simulink model "Generated_Trajectory_Linear_System"  (R2020b)
settings: Solver=VariableStepAuto  StartTime=0.0  StopTime=t_sim  RelTol=1e-3
undefined symbols (not defined in the file): A1_sim, B1_sim, Beta0Vec1_sim, OL_Traj_Gain, omega_sim, r_sim
settings Model: Creator=domin  LastModifiedBy=domin

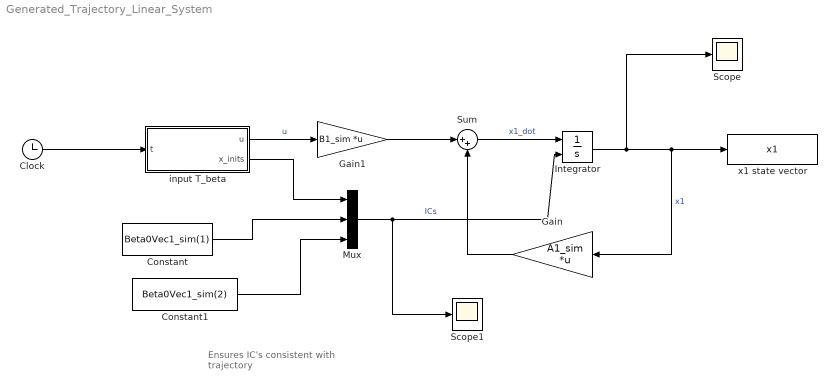
== system Generated_Trajectory_Linear_System ==
  note: Ensures IC's consistent with trajectory
  Clock : Clock
  Constant : Constant  Value=Beta0Vec1_sim(1)
  Constant1 : Constant  Value=Beta0Vec1_sim(2)
  Gain : Gain  Gain=A1_sim  Multiplication=Matrix(K*u)
  Gain1 : Gain  Gain=B1_sim  Multiplication=Matrix(K*u)
  Integrator : Integrator  InitialConditionSource=external
  Mux : Mux  Inputs=3
  Scope : Scope
  Scope1 : Scope
  Sum : Sum  Inputs=|++
  input T_beta : Subsystem
  x1 state vector : ToWorkspace  VariableName=x1  SampleTime=-1
  wires:
  Clock/1 -> input T_beta/1(t)
  Sum/1 -> Integrator/1  "x1_dot"
  Integrator/1 -> Scope/1, Gain/1, x1 state vector/1  "x1"
  input T_beta/1(u) -> Gain1/1  "u"
  Gain1/1 -> Sum/1
  Gain/1 -> Sum/2
  Constant1/1 -> Mux/3
  Constant/1 -> Mux/2
  input T_beta/2(x_inits) -> Mux/1
  Mux/1 -> Scope1/1, Integrator/2  "ICs"

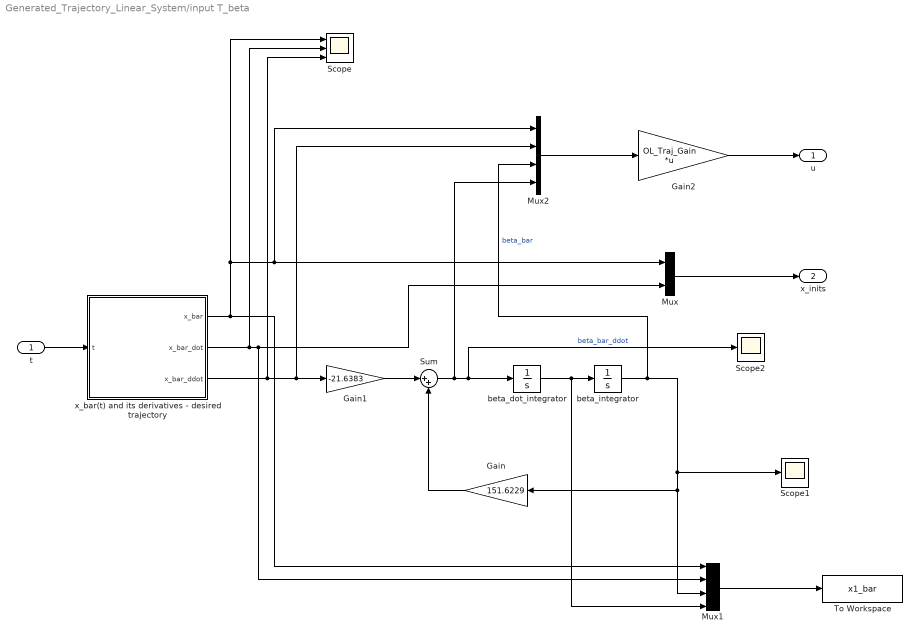
== system Generated_Trajectory_Linear_System/input T_beta ==
  t : Inport
  Gain : Gain  Gain=151.6229
  Gain1 : Gain  Gain=-21.6383
  Gain2 : Gain  Gain=OL_Traj_Gain  Multiplication=Matrix(K*u)
  Mux : Mux  Inputs=2
  Mux1 : Mux
  Mux2 : Mux
  Scope : Scope  NumInputPorts=3
  Scope1 : Scope
  Scope2 : Scope
  Sum : Sum  Inputs=|++
  To Workspace : ToWorkspace  VariableName=x1_bar  SampleTime=-1
  beta_dot_integrator : Integrator  InitialCondition=Beta0Vec1_sim(2)
  beta_integrator : Integrator  InitialCondition=Beta0Vec1_sim(1)
  x_bar(t) and its derivatives - desired trajectory : MATLAB Function  TreatAsAtomicUnit=on
  u : Outport
  x_inits : Outport  Port=2
  wires:
  t/1 -> x_bar(t) and its derivatives - desired trajectory/1(t)
  Sum/1 -> Mux2/4, Scope2/1, beta_dot_integrator/1  "beta_bar_ddot"
  beta_dot_integrator/1 -> Mux1/4, beta_integrator/1
  beta_integrator/1 -> Mux2/3, Mux1/3, Gain/1, Scope1/1  "beta_bar"
  Gain/1 -> Sum/2
  x_bar(t) and its derivatives - desired trajectory/3(x_bar_ddot) -> Scope/3, Mux2/2, Gain1/1
  Gain1/1 -> Sum/1
  x_bar(t) and its derivatives - desired trajectory/1(x_bar) -> Mux1/1, Mux2/1, Mux/1, Scope/1
  x_bar(t) and its derivatives - desired trajectory/2(x_bar_dot) -> Scope/2, Mux1/2, Mux/2
  Mux/1 -> x_inits/1
  Mux1/1 -> To Workspace/1
  Gain2/1 -> u/1
  Mux2/1 -> Gain2/1

== matlab function Generated_Trajectory_Linear_System/input T_beta/x_bar(t) and its derivatives - desired trajectory ==
  data: t input; x_bar output; x_bar_dot output; x_bar_ddot output; r_sim parameter; omega_sim parameter
function [x_bar,x_bar_dot,x_bar_ddot] = fcn(t,r_sim, omega_sim)

w = omega_sim;
r = r_sim;

x_bar = r*cos(w*t);
x_bar_dot = -r*w*sin(w*t);
x_bar_ddot = -r*w^2*cos(w*t);
